simulink model "arm_sampling"  (R2024b)
settings: Solver=VariableStepAuto  StartTime=0.0  StopTime=1000  RelTol=1e-3
libraries: models_lib x1
settings Model: Creator=ikostelidis  LastModifiedBy=ikostelidis

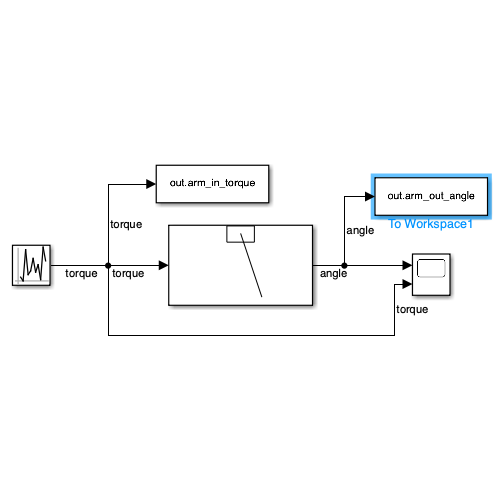
[thumbnail: Simulink's stored preview of the top-level diagram]
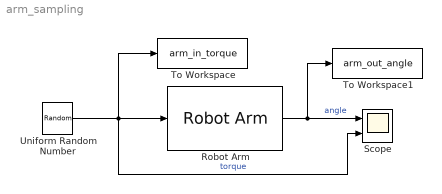
== system arm_sampling ==
  Robot Arm : models_lib/Robot Arm  SystemSampleTime=-1  VariantActivationTime=update diagram  AllowFlexibleInterface=on  Latency=0  AutoFrameSizeCalculation=off
  Scope : Scope  NumInputPorts=2
  To Workspace : ToWorkspace  VariableName=arm_in_torque  SampleTime=0.1
      settings: Save2DSignal=2-D array (concatenate along first dimension)
  To Workspace1 : ToWorkspace  VariableName=arm_out_angle  SampleTime=0.1
      settings: Save2DSignal=2-D array (concatenate along first dimension)
  Uniform Random Number : UniformRandomNumber  Minimum=-4  Maximum=4  SampleTime=2
  wires:
  Uniform Random Number/1 -> Robot Arm/1, Scope/2, To Workspace/1  "torque"
  Robot Arm/1 -> To Workspace1/1, Scope/1  "angle"
